simulink model "networkstate"  (R2025a)
settings: Solver=VariableStepAuto  StartTime=0.0  StopTime=10.0  RelTol=1e-3
settings Model: Creator=sz-p1367  LastModifiedBy=sz-p1367

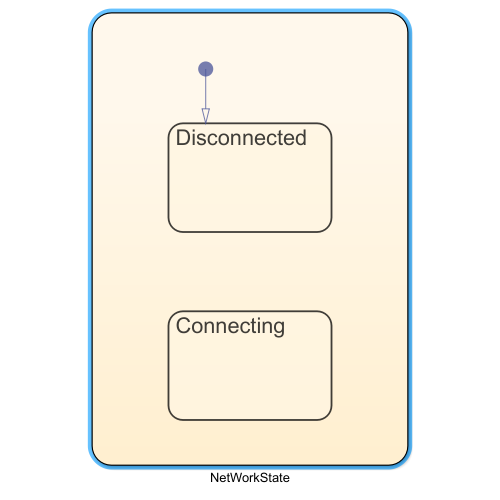
[thumbnail: Simulink's stored preview of the top-level diagram]
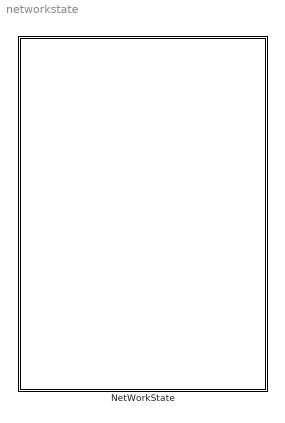
== system networkstate ==
  NetWorkState : Stateflow chart  TreatAsAtomicUnit=on

== stateflow chart networkstate/NetWorkState ==
  state Init
  state Disconnected
  state Connecting
  state Reconnecting
  state Connected
  (default) -> Init
  Init -> Disconnected
  Connected -> Disconnected
  Reconnecting -> Disconnected [order 1]
  Disconnected -> Connecting
  Connecting -> Disconnected [order 1]
  Connecting -> Reconnecting [order 3]
  Connecting -> Connected [order 2]
  Reconnecting -> Connected [order 2]
